simulink model "KUKAKR70"  (R2022b)
settings: Solver=ode4  StartTime=0.0  StopTime=SimulinkSimTime  FixedStep=Ts  RelTol=1e-3
values from neighbouring files (symbols this model uses):
  X = 1200    [KR70InverseDynamics.m]
  Y = 1200    [KR70InverseDynamics.m]
  Z = 1200    [KR70InverseDynamics.m]
libraries: nesl_utility x35, sm_lib x32, simulink_extras x7, sharedtransform x1
settings Model: Creator=Aboudi  LastModifiedBy=revdu
settings SolverCC: AlgebraicLoopSolver=TrustRegion
settings OptimizationCC: EnhancedBackFolding=on  PassReuseOutputArgsAs=Individual arguments  ZeroExternalMemoryAtStartup=off  ZeroInternalMemoryAtStartup=off  MaxStackSize=64  OptimizeBlockOrder=speed  DifferentSizesBufferReuse=on  OptimizationCustomize=off  EfficientTunableParamExpr=on
settings DebuggingCC: ParameterTunabilityLossMsg=error  UnconnectedInputMsg=warning  UnconnectedOutputMsg=warning  UnconnectedLineMsg=warning  SFMachineParentedDataDiag=warning
settings HardwareCC: ProdBitPerPointer=32  ProdBitPerSizeT=32  ProdBitPerPtrDiffT=32  ProdLargestAtomicFloat=None  ProdIntDivRoundTo=Undefined  ProdEndianess=Unspecified  ProdWordSize=32  ProdHWDeviceType=Generic->Unspecified (assume 32-bit Generic)
settings ModelReferenceCC: EnableRefExpFcnMdlSchedulingChecks=on
settings SFSimCC: MATLABDynamicMemAlloc=off
settings RTWCC: Description=Embedded Coder  SystemTargetFile=ert.tlc  HardwareBoard=Robot Operating System (ROS)  TLCOptions="-aInlineSetEventsForThisBaseRateFcn=TLC_FALSE -aSuppressMultiTaskScheduler=TLC_FALSE  -aRateBasedStepFcn=0"  TemplateMakefile=ert_default_tmf  Toolchain=Catkin  TargetLang=C++
settings CodeAppCC: ForceParamTrailComments=on  IgnoreCustomStorageClasses=off  OperatorAnnotations=on  SimulinkDataObjDesc=on  SFDataObjDesc=on  InsertBlockDesc=on
settings ExplorerConfigSet: InternalSimMechanicsExplorerSettings="<ExplorerConfiguration><canonicalview>aerospace</canonicalview><AnimationSetting><BasePlaybackSpeed>1.0</BasePlaybackSpeed><PlaybackSpeedFactor>1.0</PlaybackSpeedFactor></AnimationSetting><TilePanel><TileInfo><Tiles Columns=\"1\" Count=\"1\" Rows=\"1\"><Column Weight=\"1\"/><Row Weight=\"1\"/><Tile Height=\"1\" Width=\"1\" X=\"0\" Y=\"0\"/></Tiles></TileInfo><SceneInfo><SceneViewer><BGColor><R>0.60000002384185791</R><G>0.60000002384185791</G><B>0.60000002384185791</B></BGColor><Camera><DoPerspective>off</DoPerspective><Position><X>5.06313439550906796</X><Y>0.0784860108113666355</Y><Z>2.80097645569289577</Z></Position><Center><X>0.122639400059972203</X><Y>0.384687639263078585</Y><Z>0.502344850293265921</Z></Center><Up><X>-0.42040582822240502</X><Y>0.0254642749424247583</Y><Z>0.906978781614151353</Z></Up><ViewLimDist>1</ViewLimDist><YLim>1.2254397847778391</YLim><XLim>1.82716918582345955</XLim></Camera></SceneViewer></SceneInfo></TilePanel><MechEditorPanel><Cameras/><GfxPanelCameraMap/><VideoCreator><PlaybackSpeedRatio>1.0</PlaybackSpeedRatio><FrameRate>30</FrameRate><VideoFormat>Motion JPEG AVI</VideoFormat><FrameSize>auto</FrameSize></VideoCreator></MechEditorPanel></ExplorerConfiguration>"

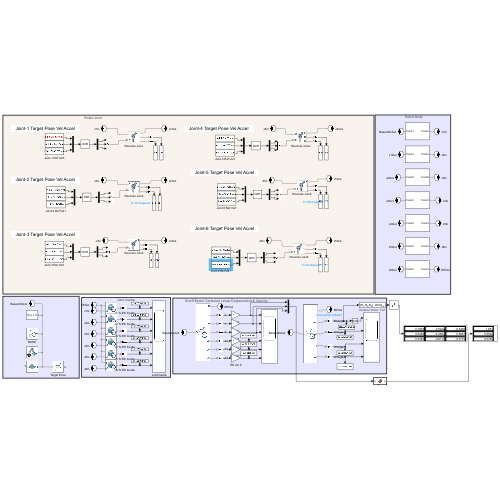
[thumbnail: Simulink's stored preview of the top-level diagram]
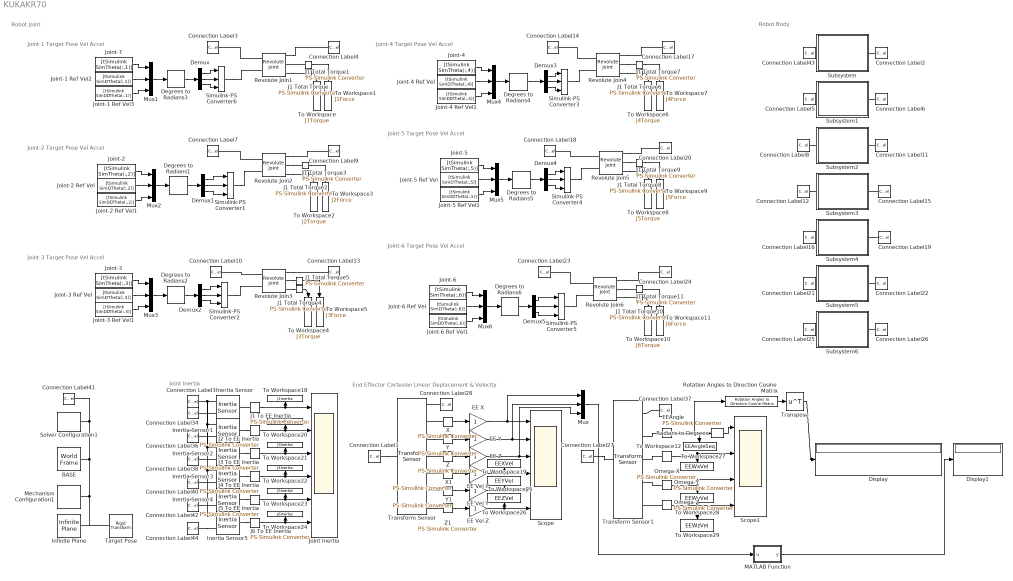
== system KUKAKR70 ==
  note: Robot Body
  note: Robot Joint
  note: Joint-1 Target Pose Vel Accel
  note: Joint-2 Target Pose Vel Accel
  note: Joint-3 Target Pose Vel Accel
  note: Joint-4 Target Pose Vel Accel
  note: Joint-5 Target Pose Vel Accel
  note: Joint-6 Target Pose Vel Accel
  note: Joint Inertia
  note: End Effector Cartesian Linear Deplacement & Velocity
  BASE : sm_lib/Frames and Transforms/World Frame
  Connection Label{1,27,41,43} (4 alike) : ConnectionLabel  Label=BasetoRobot
  Connection Label10 : ConnectionLabel  Label=J3In
  Connection Label11 : ConnectionLabel  Label=J3In
  Connection Label12 : ConnectionLabel  Label=J3Out
  Connection Label13 : ConnectionLabel  Label=J3Out
  Connection Label14 : ConnectionLabel  Label=J4In
  Connection Label15 : ConnectionLabel  Label=J4In
  Connection Label16 : ConnectionLabel  Label=J4Out
  Connection Label17 : ConnectionLabel  Label=J4Out
  Connection Label18 : ConnectionLabel  Label=J5In
  Connection Label19 : ConnectionLabel  Label=J5In
  Connection Label2 : ConnectionLabel  Label=J1In
  Connection Label20 : ConnectionLabel  Label=J5Out
  Connection Label21 : ConnectionLabel  Label=J5Out
  Connection Label22 : ConnectionLabel  Label=J6In
  Connection Label23 : ConnectionLabel  Label=J6In
  Connection Label24 : ConnectionLabel  Label=J6Out
  Connection Label25 : ConnectionLabel  Label=J6Out
  Connection Label{26,28,33,37} (4 alike) : ConnectionLabel  Label=EEOut
  Connection Label3 : ConnectionLabel  Label=J1In
  Connection Label34 : ConnectionLabel  Label=J1In
  Connection Label36 : ConnectionLabel  Label=J2In
  Connection Label38 : ConnectionLabel  Label=J3In
  Connection Label4 : ConnectionLabel  Label=J1Out
  Connection Label40 : ConnectionLabel  Label=J4In
  Connection Label42 : ConnectionLabel  Label=J5In
  Connection Label44 : ConnectionLabel  Label=J6In
  Connection Label5 : ConnectionLabel  Label=J1Out
  Connection Label6 : ConnectionLabel  Label=J2In
  Connection Label7 : ConnectionLabel  Label=J2In
  Connection Label8 : ConnectionLabel  Label=J2Out
  Connection Label9 : ConnectionLabel  Label=J2Out
  Degrees to Radians{1..6} (6 alike) : simulink_extras/Transformations/Degrees to Radians
  Demux{,1..5} (6 alike) : Demux  Outputs=3
  Display : Display
  Display1 : Display
  EE Vel X : Gain
  EE Vel Y : Gain
  EE Vel Z : Gain
  EE X : Gain
  EE Y : Gain
  EE Z : Gain
  EEAngle : nesl_utility/PS-Simulink Converter  PhysicalDomain=network_engine_domain  SubClassName=ps_output  LeftPortType=input  RightPortType=output  PseudoPeriodic=off  Frequencies=[]  VectorFormat=1-D array  Unit=rad  AffineConversion=off
  Inertia Sensor : sm_lib/Body Elements/Inertia Sensor  SensorExtent=BodyGroup  SpanWeldJoints=off  ExcludeGroundedBodies=off  MeasurementFrame=Custom  SenseMass=off  SenseCenterOfMass=off  SenseInertiaMatrix=on  SenseCenteredInertiaMatrix=off  SensePrincipalInertiaMatrix=off  SenseRotationMatrix=off  GraphicType=None  PrincipalInertiaFrameSize=20  GraphicVisPropType=SimpleVisualProperties  GraphicDiffuseColor=[1.0 1.0 0.0]  GraphicSpecularColor=[0.5 0.5 0.5 1.0]  GraphicAmbientColor=[0.15 0.15 0.15 1.0]  GraphicEmissiveColor=[0.0 0.0 0.0 1.0]  GraphicShininess=75  GraphicOpacity=0
  Inertia Sensor1 : sm_lib/Body Elements/Inertia Sensor  SensorExtent=BodyGroup  SpanWeldJoints=on  ExcludeGroundedBodies=off  MeasurementFrame=Custom  SenseMass=off  SenseCenterOfMass=off  SenseInertiaMatrix=on  SenseCenteredInertiaMatrix=off  SensePrincipalInertiaMatrix=off  SenseRotationMatrix=off  GraphicType=None  PrincipalInertiaFrameSize=20  GraphicVisPropType=SimpleVisualProperties  GraphicDiffuseColor=[1.0 1.0 0.0]  GraphicSpecularColor=[0.5 0.5 0.5 1.0]  GraphicAmbientColor=[0.15 0.15 0.15 1.0]  GraphicEmissiveColor=[0.0 0.0 0.0 1.0]  GraphicShininess=75  GraphicOpacity=1.0
  Inertia Sensor{2..5} (4 alike) : sm_lib/Body Elements/Inertia Sensor  SensorExtent=BodyGroup  SpanWeldJoints=off  ExcludeGroundedBodies=off  MeasurementFrame=Custom  SenseMass=off  SenseCenterOfMass=off  SenseInertiaMatrix=on  SenseCenteredInertiaMatrix=off  SensePrincipalInertiaMatrix=off  SenseRotationMatrix=off  GraphicType=None  PrincipalInertiaFrameSize=20  GraphicVisPropType=SimpleVisualProperties  GraphicDiffuseColor=[1.0 1.0 0.0]  GraphicSpecularColor=[0.5 0.5 0.5 1.0]  GraphicAmbientColor=[0.15 0.15 0.15 1.0]  GraphicEmissiveColor=[0.0 0.0 0.0 1.0]  GraphicShininess=75  GraphicOpacity=1.0
  Infinite Plane : sm_lib/Curves and Surfaces/Infinite Plane  GraphicType=Rectangle  GraphicPlaneWidth=5  GraphicPlaneWidthUnits=m  GraphicPlaneHeight=5  GraphicPlaneHeightUnits=m  GraphicVisPropType=SimpleVisualProperties  GraphicDiffuseColor=[1 0 0]  GraphicOpacity=.25  GraphicSpecularColor=[0.5 0.5 0.5 1.0]  GraphicAmbientColor=[0.15 0.15 0.15 1.0]  GraphicEmissiveColor=[0.0 0.0 0.0 1.0]  GraphicShininess=75
  J1 To EE Inertia : nesl_utility/PS-Simulink Converter  PhysicalDomain=network_engine_domain  SubClassName=ps_output  LeftPortType=input  RightPortType=output  PseudoPeriodic=off  Frequencies=[]  VectorFormat=1-D array  Unit=inherit  AffineConversion=off
  J1 Total Torque{,2,4,6,8,10} (6 alike) : nesl_utility/PS-Simulink Converter  PhysicalDomain=network_engine_domain  SubClassName=ps_output  LeftPortType=input  RightPortType=output  PseudoPeriodic=off  Frequencies=[]  VectorFormat=1-D array  Unit=N*m  AffineConversion=off
  J1 Total Torque{1,3,5,7,9,11} (6 alike) : nesl_utility/PS-Simulink Converter  PhysicalDomain=network_engine_domain  SubClassName=ps_output  LeftPortType=input  RightPortType=output  PseudoPeriodic=off  Frequencies=[]  VectorFormat=1-D array  Unit=N  AffineConversion=off
  J2 To EE Inertia : nesl_utility/PS-Simulink Converter  PhysicalDomain=network_engine_domain  SubClassName=ps_output  LeftPortType=input  RightPortType=output  PseudoPeriodic=off  Frequencies=[]  VectorFormat=1-D array  Unit=inherit  AffineConversion=off
  J3 To EE Inertia : nesl_utility/PS-Simulink Converter  PhysicalDomain=network_engine_domain  SubClassName=ps_output  LeftPortType=input  RightPortType=output  PseudoPeriodic=off  Frequencies=[]  VectorFormat=1-D array  Unit=inherit  AffineConversion=off
  J4 To EE Inertia : nesl_utility/PS-Simulink Converter  PhysicalDomain=network_engine_domain  SubClassName=ps_output  LeftPortType=input  RightPortType=output  PseudoPeriodic=off  Frequencies=[]  VectorFormat=1-D array  Unit=inherit  AffineConversion=off
  J5 To EE Inertia : nesl_utility/PS-Simulink Converter  PhysicalDomain=network_engine_domain  SubClassName=ps_output  LeftPortType=input  RightPortType=output  PseudoPeriodic=off  Frequencies=[]  VectorFormat=1-D array  Unit=inherit  AffineConversion=off
  J6 To EE Inertia : nesl_utility/PS-Simulink Converter  PhysicalDomain=network_engine_domain  SubClassName=ps_output  LeftPortType=input  RightPortType=output  PseudoPeriodic=off  Frequencies=[]  VectorFormat=1-D array  Unit=inherit  AffineConversion=off
  Joint Inertia : Scope  NumInputPorts=6
  Joint-1 Ref Vel2 : FromWorkspace  VariableName=[tSimulink SimDTheta(:,1)]  SampleTime=-1  OutputAfterFinalValue=Holding final value
  Joint-1 Ref Vel3 : FromWorkspace  VariableName=[tSimulink SimDDTheta(:,1)]  SampleTime=-1  OutputAfterFinalValue=Holding final value
  Joint-2 : FromWorkspace  VariableName=[tSimulink SimTheta(:,2)]  SampleTime=-1  OutputAfterFinalValue=Holding final value
  Joint-2 Ref Vel : FromWorkspace  VariableName=[tSimulink SimDTheta(:,2)]  SampleTime=-1  OutputAfterFinalValue=Holding final value
  Joint-2 Ref Vel1 : FromWorkspace  VariableName=[tSimulink SimDDTheta(:,2)]  SampleTime=-1  OutputAfterFinalValue=Holding final value
  Joint-3 : FromWorkspace  VariableName=[tSimulink SimTheta(:,3)]  SampleTime=-1  OutputAfterFinalValue=Holding final value
  Joint-3 Ref Vel : FromWorkspace  VariableName=[tSimulink SimDTheta(:,3)]  SampleTime=-1  OutputAfterFinalValue=Holding final value
  Joint-3 Ref Vel1 : FromWorkspace  VariableName=[tSimulink SimDDTheta(:,3)]  SampleTime=-1  OutputAfterFinalValue=Holding final value
  Joint-4 : FromWorkspace  VariableName=[tSimulink SimTheta(:,4)]  SampleTime=-1  OutputAfterFinalValue=Holding final value
  Joint-4 Ref Vel : FromWorkspace  VariableName=[tSimulink SimDTheta(:,4)]  SampleTime=-1  OutputAfterFinalValue=Holding final value
  Joint-4 Ref Vel1 : FromWorkspace  VariableName=[tSimulink SimDDTheta(:,4)]  SampleTime=-1  OutputAfterFinalValue=Holding final value
  Joint-5 : FromWorkspace  VariableName=[tSimulink SimTheta(:,5)]  SampleTime=-1  OutputAfterFinalValue=Holding final value
  Joint-5 Ref Vel : FromWorkspace  VariableName=[tSimulink SimDTheta(:,5)]  SampleTime=-1  OutputAfterFinalValue=Holding final value
  Joint-5 Ref Vel1 : FromWorkspace  VariableName=[tSimulink SimDDTheta(:,5)]  SampleTime=-1  OutputAfterFinalValue=Holding final value
  Joint-6 : FromWorkspace  VariableName=[tSimulink SimTheta(:,6)]  SampleTime=-1  OutputAfterFinalValue=Holding final value
  Joint-6 Ref Vel : FromWorkspace  VariableName=[tSimulink SimDTheta(:,6)]  SampleTime=-1  OutputAfterFinalValue=Holding final value
  Joint-6 Ref Vel1 : FromWorkspace  VariableName=[tSimulink SimDDTheta(:,6)]  SampleTime=-1  OutputAfterFinalValue=Holding final value
  Joint-7 : FromWorkspace  VariableName=[tSimulink SimTheta(:,1)]  SampleTime=-1  OutputAfterFinalValue=Holding final value
  MATLAB Function : MATLAB Function  TreatAsAtomicUnit=on
  Mechanism Configuration1 : sm_lib/Utilities/Mechanism Configuration  UniformGravity=Constant  GravityVector=[0 0 -9.80665]  GravityUnits=m/s^2  LinearizationDelta=0.001  JointModeTransitionNonlinearIterations=2
  Mux{,1..6} (7 alike) : Mux  Inputs=3
  Omega-X : nesl_utility/PS-Simulink Converter  PhysicalDomain=network_engine_domain  SubClassName=ps_output  LeftPortType=input  RightPortType=output  PseudoPeriodic=off  Frequencies=[]  VectorFormat=1-D array  Unit=rad/s  AffineConversion=off
  Omega-Y : nesl_utility/PS-Simulink Converter  PhysicalDomain=network_engine_domain  SubClassName=ps_output  LeftPortType=input  RightPortType=output  PseudoPeriodic=off  Frequencies=[]  VectorFormat=1-D array  Unit=rad/s  AffineConversion=off
  Omega-Z : nesl_utility/PS-Simulink Converter  PhysicalDomain=network_engine_domain  SubClassName=ps_output  LeftPortType=input  RightPortType=output  PseudoPeriodic=off  Frequencies=[]  VectorFormat=1-D array  Unit=rad/s  AffineConversion=off
  Radians to Degrees : simulink_extras/Transformations/Radians to Degrees
  Revolute Join{1..6} (6 alike) : sm_lib/Joints/Revolute Joint  JointMode=Normal  SenseConstraintForce=off  SenseConstraintForceX=off  SenseConstraintForceY=off  SenseConstraintForceZ=off  SenseConstraintTorque=off  SenseConstraintTorqueX=off  SenseConstraintTorqueY=off  SenseConstraintTorqueZ=off  SenseTotalForce=on  SenseTotalForceX=off  SenseTotalForceY=off  SenseTotalForceZ=off  SenseTotalTorque=on  SenseTotalTorqueX=off  SenseTotalTorqueY=off  SenseTotalTorqueZ=off  CompositeWrenchDir=FollowerOnBase  CompositeWrenchFrame=FollowerFrame  EquilibriumPosition=0  EquilibriumPositionUnits=deg  SpringStiffness=0  SpringStiffnessUnits=N*m/deg  DampingCoefficient=0  DampingCoefficientUnits=N*m/(deg/s)  TorqueActuationMode=ComputedTorque  MotionActuationMode=InputMotion  SensePosition=off  SenseVelocity=off  SenseAcceleration=off  SenseTorqueForce=off  SenseLowerLimitTorqueForce=off  SenseUpperLimitTorqueForce=off  LowerLimitSpecify=off  LowerLimitBound=-90  LowerLimitBoundUnits=deg  LowerLimitStiffness=1e4  LowerLimitStiffnessUnits=N*m/deg  LowerLimitDamping=10  LowerLimitDampingUnits=N*m/(deg/s)  LowerLimitTransitionRegionWidth=0.1  LowerLimitTransitionRegionWidthUnits=deg  UpperLimitSpecify=off  UpperLimitBound=90  UpperLimitBoundUnits=deg  UpperLimitStiffness=1e4  UpperLimitStiffnessUnits=N*m/deg  UpperLimitDamping=10  UpperLimitDampingUnits=N*m/(deg/s)  UpperLimitTransitionRegionWidth=0.1  UpperLimitTransitionRegionWidthUnits=deg  PositionTargetSpecify=off  PositionTargetPriority=High  PositionTargetValue=0  PositionTargetValueUnits=deg  VelocityTargetSpecify=off  VelocityTargetPriority=High  VelocityTargetValue=0  VelocityTargetValueUnits=deg/s
  Rotation Angles to Direction Cosine Matrix : sharedtransform/Rotation Angles to Direction Cosine Matrix  rotationOrder=XYZ  aMode=aMode
  Scope : Scope  NumInputPorts=6
  Scope1 : Scope  NumInputPorts=4
  Simulink-PS Converter{1..6} (6 alike) : nesl_utility/Simulink-PS Converter  PhysicalDomain=network_engine_domain  SubClassName=ps_input  LeftPortType=input  RightPortType=output  PseudoPeriodic=off  Frequencies=[]  NoiseDistribution=none  NoiseParameters=[]  Unit=1  AffineConversion=off  FilteringAndDerivatives=provide  SimscapeFilterOrder=2  InputFilterTimeConstant=Ts  UdotUserProvided=2
  Solver Configuration1 : nesl_utility/Solver Configuration  PhysicalDomain=network_engine_domain  SubClassName=solver  LeftPortType=input  RightPortType=generic  Tones=[]  Harmonics=[]  SimulateNoise=off  Profile=off  UseLocalSampling=off  EnableSwitchedLinearOptims=on  FrequencyDomain=off  UseCCode=off  RelTol=0.001  AbsTol=1e-06  MinStep=1e-09  ToWorkspace=off  RevertToSquareIcSolve=off  NumHomotopyIterations=100  PhasorMode=off  PhasorModeNumHarmonics=1  ConsistencySolver=NEWTON_FTOL  IndexReductionMethod=DerivativeReplacement  DoDC=off  ResidualTolerance=1e-09  ConsistencyTolSource=GLOBAL  ConsistencyAbsTol=0.001  ConsistencyRelTol=0.001  ConsistencyTolFactor=0.001  UseLocalSolver=off  LocalSolverChoice=NE_BACKWARD_EULER_ADVANCER  ResolveIndetEquations=on  FunctionEvalNumThread=1  LocalSolverSampleTime=0.001  DoFixedCost=off  MaxNonlinIter=3  MaxModeIter=2  ComputeImpulses=off  ImpulseIterations=2  LinearAlgebra=Full  LinearAlgebraNumThread=0  EquationFormulation=NE_FREQUENCY_TIME_EF  DelaysMemoryBudget=1024  AutomaticFiltering=on  FilteringTimeConstant=0.001  PartitionStorageMethod=AS_NEEDED  PartitionMemoryBudget=1024  PartitionMethod=FAST
  Subsystem : Subsystem
  Subsystem1 : Subsystem
  Subsystem2 : Subsystem
  Subsystem3 : Subsystem
  Subsystem4 : Subsystem
  Subsystem5 : Subsystem
  Subsystem6 : Subsystem
  Target Pose : sm_lib/Frames and Transforms/Rigid Transform  TranslationMethod=Cartesian  TranslationStandardOffset=0  TranslationLengthUnit=mm  TranslationStandardAxis=+Z  TranslationCartesianOffset=AllTargetPose(1:3,4,end)  TranslationROffset=0  TranslationROffsetUnits=m  TranslationZOffset=0  TranslationZOffsetUnits=m  TranslationThetaOffset=0  TranslationThetaOffsetUnits=deg  RotationMethod=RotationMatrix  RotationAngleUnits=deg  RotationStandardAxis=+Z  RotationAngle=0.0  RotationArbitraryAxis=[0 0 1]  FollAlignAxisA=+X  BaseAlignAxisA=+Y  FollAlignAxisB=+Y  BaseAlignAxisB=+Z  RotationSequenceAxes=FollowerAxes  RotationSequence=XYX  RotationSequenceAngles=[0 0 0]  RotationSequenceAnglesUnits=deg  RotationMatrix=AllTargetPose(1:3,1:3,end)  Quaternion=[1 0 0 0]
  To Workspace : ToWorkspace  VariableName=J1Torque  SaveFormat=Timeseries  SampleTime=-1
  To Workspace1 : ToWorkspace  VariableName=J1Force  SaveFormat=Timeseries  SampleTime=-1
  To Workspace10 : ToWorkspace  VariableName=J6Torque  SaveFormat=Timeseries  SampleTime=-1
  To Workspace11 : ToWorkspace  VariableName=J6Force  SaveFormat=Timeseries  SampleTime=-1
  To Workspace12 : ToWorkspace  VariableName=EEAngleSeq  SaveFormat=Timeseries  SampleTime=-1
  To Workspace18 : ToWorkspace  VariableName=J1Inertia  SaveFormat=Timeseries  SampleTime=-1
  To Workspace19 : ToWorkspace  VariableName=EEXVel  SaveFormat=Timeseries  SampleTime=-1
  To Workspace2 : ToWorkspace  VariableName=J2Torque  SaveFormat=Timeseries  SampleTime=-1
  To Workspace20 : ToWorkspace  VariableName=J2Inertia  SaveFormat=Timeseries  SampleTime=-1
  To Workspace21 : ToWorkspace  VariableName=J3Inertia  SaveFormat=Timeseries  SampleTime=-1
  To Workspace22 : ToWorkspace  VariableName=J4Inertia  SaveFormat=Timeseries  SampleTime=-1
  To Workspace23 : ToWorkspace  VariableName=J5Inertia  SaveFormat=Timeseries  SampleTime=-1
  To Workspace24 : ToWorkspace  VariableName=J6Inertia  SaveFormat=Timeseries  SampleTime=-1
  To Workspace25 : ToWorkspace  VariableName=EEYVel  SaveFormat=Timeseries  SampleTime=-1
  To Workspace26 : ToWorkspace  VariableName=EEZVel  SaveFormat=Timeseries  SampleTime=-1
  To Workspace27 : ToWorkspace  VariableName=EEWxVel  SaveFormat=Timeseries  SampleTime=-1
  To Workspace28 : ToWorkspace  VariableName=EEWyVel  SaveFormat=Timeseries  SampleTime=-1
  To Workspace29 : ToWorkspace  VariableName=EEWzVel  SaveFormat=Timeseries  SampleTime=-1
  To Workspace3 : ToWorkspace  VariableName=J2Force  SaveFormat=Timeseries  SampleTime=-1
  To Workspace4 : ToWorkspace  VariableName=J3Torque  SaveFormat=Timeseries  SampleTime=-1
  To Workspace5 : ToWorkspace  VariableName=J3Force  SaveFormat=Timeseries  SampleTime=-1
  To Workspace6 : ToWorkspace  VariableName=J4Torque  SaveFormat=Timeseries  SampleTime=-1
  To Workspace7 : ToWorkspace  VariableName=J4Force  SaveFormat=Timeseries  SampleTime=-1
  To Workspace8 : ToWorkspace  VariableName=J5Torque  SaveFormat=Timeseries  SampleTime=-1
  To Workspace9 : ToWorkspace  VariableName=J5Force  SaveFormat=Timeseries  SampleTime=-1
  Transform Sensor : sm_lib/Frames and Transforms/Transform Sensor  MeasurementFrame=World  SenseAngle=off  SenseAxis=off  SenseQ=off  SenseR=off  SenseRotationSequence=off  RotationSequence=XYX  SenseOmegaX=off  SenseOmegaY=off  SenseOmegaZ=off  SenseQDot=off  SenseRDot=off  SenseAlphaX=off  SenseAlphaY=off  SenseAlphaZ=off  SenseQDDot=off  SenseRDDot=off  SenseX=on  SenseY=on  SenseZ=on  SenseRad=off  SenseAzim=off  SenseDist=off  SenseInc=off  SenseXDot=on  SenseYDot=on  SenseZDot=on  SenseRadDot=off  SenseAzimDot=off  SenseDistDot=off  SenseIncDot=off  SenseXDDot=off  SenseYDDot=off  SenseZDDot=off  SenseRadDDot=off  SenseAzimDDot=off  SenseDistDDot=off  SenseIncDDot=off
  Transform Sensor1 : sm_lib/Frames and Transforms/Transform Sensor  MeasurementFrame=World  SenseAngle=off  SenseAxis=off  SenseQ=off  SenseR=off  SenseRotationSequence=on  RotationSequence=XYZ  SenseOmegaX=on  SenseOmegaY=on  SenseOmegaZ=on  SenseQDot=off  SenseRDot=off  SenseAlphaX=off  SenseAlphaY=off  SenseAlphaZ=off  SenseQDDot=off  SenseRDDot=off  SenseX=off  SenseY=off  SenseZ=off  SenseRad=off  SenseAzim=off  SenseDist=off  SenseInc=off  SenseXDot=off  SenseYDot=off  SenseZDot=off  SenseRadDot=off  SenseAzimDot=off  SenseDistDot=off  SenseIncDot=off  SenseXDDot=off  SenseYDDot=off  SenseZDDot=off  SenseRadDDot=off  SenseAzimDDot=off  SenseDistDDot=off  SenseIncDDot=off
  Transpose : Math  Operator=transpose
  X : nesl_utility/PS-Simulink Converter  PhysicalDomain=network_engine_domain  SubClassName=ps_output  LeftPortType=input  RightPortType=output  PseudoPeriodic=off  Frequencies=[]  VectorFormat=1-D array  Unit=m  AffineConversion=off
  X1 : nesl_utility/PS-Simulink Converter  PhysicalDomain=network_engine_domain  SubClassName=ps_output  LeftPortType=input  RightPortType=output  PseudoPeriodic=off  Frequencies=[]  VectorFormat=1-D array  Unit=m/s  AffineConversion=off
  Y : nesl_utility/PS-Simulink Converter  PhysicalDomain=network_engine_domain  SubClassName=ps_output  LeftPortType=input  RightPortType=output  PseudoPeriodic=off  Frequencies=[]  VectorFormat=1-D array  Unit=m  AffineConversion=off
  Y1 : nesl_utility/PS-Simulink Converter  PhysicalDomain=network_engine_domain  SubClassName=ps_output  LeftPortType=input  RightPortType=output  PseudoPeriodic=off  Frequencies=[]  VectorFormat=1-D array  Unit=m/s  AffineConversion=off
  Z : nesl_utility/PS-Simulink Converter  PhysicalDomain=network_engine_domain  SubClassName=ps_output  LeftPortType=input  RightPortType=output  PseudoPeriodic=off  Frequencies=[]  VectorFormat=1-D array  Unit=m  AffineConversion=off
  Z1 : nesl_utility/PS-Simulink Converter  PhysicalDomain=network_engine_domain  SubClassName=ps_output  LeftPortType=input  RightPortType=output  PseudoPeriodic=off  Frequencies=[]  VectorFormat=1-D array  Unit=m/s  AffineConversion=off
  wires:
  Joint-1 Ref Vel2/1 -> Mux1/2
  Joint-7/1 -> Mux1/1
  Joint-1 Ref Vel3/1 -> Mux1/3
  Mux1/1 -> Degrees to Radians3/1
  Degrees to Radians3/1 -> Demux/1
  Demux/1 -> Simulink-PS Converter6/1
  Demux/2 -> Simulink-PS Converter6/2
  Demux/3 -> Simulink-PS Converter6/3
  Demux1/3 -> Simulink-PS Converter1/3
  Demux1/2 -> Simulink-PS Converter1/2
  Demux1/1 -> Simulink-PS Converter1/1
  Degrees to Radians1/1 -> Demux1/1
  Mux2/1 -> Degrees to Radians1/1
  Joint-2 Ref Vel1/1 -> Mux2/3
  Joint-2/1 -> Mux2/1
  Joint-2 Ref Vel/1 -> Mux2/2
  Joint-3 Ref Vel/1 -> Mux3/2
  Joint-3/1 -> Mux3/1
  Joint-3 Ref Vel1/1 -> Mux3/3
  Mux3/1 -> Degrees to Radians2/1
  Degrees to Radians2/1 -> Demux2/1
  Demux2/1 -> Simulink-PS Converter2/1
  Demux2/2 -> Simulink-PS Converter2/2
  Demux2/3 -> Simulink-PS Converter2/3
  Joint-4/1 -> Mux4/1
  Demux3/3 -> Simulink-PS Converter3/3
  Demux3/1 -> Simulink-PS Converter3/1
  Degrees to Radians4/1 -> Demux3/1
  Joint-4 Ref Vel1/1 -> Mux4/3
  Demux3/2 -> Simulink-PS Converter3/2
  Mux4/1 -> Degrees to Radians4/1
  Joint-4 Ref Vel/1 -> Mux4/2
  Demux4/3 -> Simulink-PS Converter4/3
  Demux4/2 -> Simulink-PS Converter4/2
  Demux4/1 -> Simulink-PS Converter4/1
  Degrees to Radians5/1 -> Demux4/1
  Mux5/1 -> Degrees to Radians5/1
  Joint-5 Ref Vel1/1 -> Mux5/3
  Joint-5/1 -> Mux5/1
  Joint-5 Ref Vel/1 -> Mux5/2
  Joint-6 Ref Vel/1 -> Mux6/2
  Joint-6/1 -> Mux6/1
  Joint-6 Ref Vel1/1 -> Mux6/3
  Mux6/1 -> Degrees to Radians6/1
  Degrees to Radians6/1 -> Demux5/1
  Demux5/1 -> Simulink-PS Converter5/1
  Demux5/2 -> Simulink-PS Converter5/2
  Demux5/3 -> Simulink-PS Converter5/3
  J1 Total Torque/1 -> To Workspace/1
  J1 Total Torque1/1 -> To Workspace1/1
  J1 Total Torque3/1 -> To Workspace3/1
  J1 Total Torque2/1 -> To Workspace2/1
  J1 Total Torque4/1 -> To Workspace4/1
  J1 Total Torque5/1 -> To Workspace5/1
  J1 Total Torque7/1 -> To Workspace7/1
  J1 Total Torque6/1 -> To Workspace6/1
  J1 Total Torque8/1 -> To Workspace8/1
  J1 Total Torque9/1 -> To Workspace9/1
  J1 Total Torque11/1 -> To Workspace11/1
  J1 Total Torque10/1 -> To Workspace10/1
  J2 To EE Inertia/1 -> To Workspace20/1, Joint Inertia/2
  J1 To EE Inertia/1 -> To Workspace18/1, Joint Inertia/1
  J3 To EE Inertia/1 -> To Workspace21/1, Joint Inertia/3
  J6 To EE Inertia/1 -> To Workspace24/1, Joint Inertia/6
  J5 To EE Inertia/1 -> To Workspace23/1, Joint Inertia/5
  J4 To EE Inertia/1 -> To Workspace22/1, Joint Inertia/4
  EE Vel X/1 -> Scope/4, To Workspace19/1
  EE X/1 -> Mux/1, Scope/1
  EE Vel Z/1 -> To Workspace26/1, Scope/6
  Z1/1 -> EE Vel Z/1
  Z/1 -> EE Z/1
  EE Z/1 -> Mux/3, Scope/3
  Y1/1 -> EE Vel Y/1
  EE Y/1 -> Mux/2, Scope/2
  Y/1 -> EE Y/1
  X/1 -> EE X/1
  EE Vel Y/1 -> To Workspace25/1, Scope/5
  Omega-Z/1 -> To Workspace29/1, Scope1/4
  X1/1 -> EE Vel X/1
  Omega-Y/1 -> Scope1/3, To Workspace28/1
  Omega-X/1 -> Scope1/2, To Workspace27/1
  EEAngle/1 -> Rotation Angles to Direction Cosine Matrix/1, To Workspace12/1, Radians to Degrees/1
  Radians to Degrees/1 -> Scope1/1
  Rotation Angles to Direction Cosine Matrix/1 -> Transpose/1
  Mux/1 -> MATLAB Function/1(u)
  MATLAB Function/1(y) -> Display1/1
  Transpose/1 -> Display/1
  connections:
  Mechanism Configuration1/RConn1 -- Solver Configuration1/RConn1 -- Connection Label41/LConn1 -- BASE/RConn1 -- Target Pose/LConn1 -- Infinite Plane/LConn1
  Revolute Join5/RConn1 -- Connection Label20/LConn1
  Connection Label19/LConn1 -- Subsystem4/RConn1
  Subsystem3/LConn1 -- Connection Label12/LConn1
  Connection Label25/LConn1 -- Subsystem6/LConn1
  Revolute Join2/LConn1 -- Connection Label7/LConn1
  Revolute Join3/RConn1 -- Connection Label13/LConn1
  Connection Label15/LConn1 -- Subsystem3/RConn1
  Revolute Join1/LConn1 -- Connection Label3/LConn1
  Connection Label21/LConn1 -- Subsystem5/LConn1
  Connection Label16/LConn1 -- Subsystem4/LConn1
  Revolute Join2/RConn1 -- Connection Label9/LConn1
  Revolute Join5/LConn1 -- Connection Label18/LConn1
  Connection Label5/LConn1 -- Subsystem1/LConn1
  Revolute Join6/RConn1 -- Connection Label24/LConn1
  Connection Label11/LConn1 -- Subsystem2/RConn1
  Revolute Join6/LConn1 -- Connection Label23/LConn1
  Revolute Join3/LConn1 -- Connection Label10/LConn1
  Connection Label22/LConn1 -- Subsystem5/RConn1
  Revolute Join4/LConn1 -- Connection Label14/LConn1
  Connection Label2/LConn1 -- Subsystem/RConn1
  Connection Label43/LConn1 -- Subsystem/LConn1
  Revolute Join1/RConn1 -- Connection Label4/LConn1
  Connection Label6/LConn1 -- Subsystem1/RConn1
  Subsystem2/LConn1 -- Connection Label8/LConn1
  Connection Label26/LConn1 -- Subsystem6/RConn1
  Revolute Join4/RConn1 -- Connection Label17/LConn1
  Simulink-PS Converter6/RConn1 -- Revolute Join1/LConn2
  Simulink-PS Converter1/RConn1 -- Revolute Join2/LConn2
  Simulink-PS Converter2/RConn1 -- Revolute Join3/LConn2
  Simulink-PS Converter3/RConn1 -- Revolute Join4/LConn2
  Simulink-PS Converter4/RConn1 -- Revolute Join5/LConn2
  Simulink-PS Converter5/RConn1 -- Revolute Join6/LConn2
  Revolute Join1/RConn3 -- J1 Total Torque/LConn1
  J1 Total Torque1/LConn1 -- Revolute Join1/RConn2
  Revolute Join2/RConn2 -- J1 Total Torque3/LConn1
  Revolute Join2/RConn3 -- J1 Total Torque2/LConn1
  Revolute Join3/RConn3 -- J1 Total Torque4/LConn1
  Revolute Join3/RConn2 -- J1 Total Torque5/LConn1
  Revolute Join4/RConn2 -- J1 Total Torque7/LConn1
  Revolute Join4/RConn3 -- J1 Total Torque6/LConn1
  Revolute Join5/RConn3 -- J1 Total Torque8/LConn1
  Revolute Join5/RConn2 -- J1 Total Torque9/LConn1
  Revolute Join6/RConn3 -- J1 Total Torque10/LConn1
  Revolute Join6/RConn2 -- J1 Total Torque11/LConn1
  Connection Label33/LConn1 -- Inertia Sensor1/LConn1 -- Inertia Sensor2/LConn1 -- Inertia Sensor4/LConn1 -- Inertia Sensor5/LConn1 -- Inertia Sensor3/LConn1 -- Inertia Sensor/LConn1
  Connection Label34/LConn1 -- Inertia Sensor/LConn2
  Connection Label38/LConn1 -- Inertia Sensor2/LConn2
  Inertia Sensor3/RConn1 -- J4 To EE Inertia/LConn1
  Inertia Sensor1/RConn1 -- J2 To EE Inertia/LConn1
  J1 To EE Inertia/LConn1 -- Inertia Sensor/RConn1
  Connection Label40/LConn1 -- Inertia Sensor3/LConn2
  Inertia Sensor5/RConn1 -- J6 To EE Inertia/LConn1
  Connection Label42/LConn1 -- Inertia Sensor4/LConn2
  Connection Label36/LConn1 -- Inertia Sensor1/LConn2
  Inertia Sensor4/RConn1 -- J5 To EE Inertia/LConn1
  Connection Label44/LConn1 -- Inertia Sensor5/LConn2
  Inertia Sensor2/RConn1 -- J3 To EE Inertia/LConn1
  X/LConn1 -- Transform Sensor/RConn2
  Connection Label1/LConn1 -- Transform Sensor/LConn1
  X1/LConn1 -- Transform Sensor/RConn5
  Transform Sensor/RConn3 -- Y/LConn1
  Z1/LConn1 -- Transform Sensor/RConn7
  Connection Label27/LConn1 -- Transform Sensor1/LConn1
  Z/LConn1 -- Transform Sensor/RConn4
  Y1/LConn1 -- Transform Sensor/RConn6
  Connection Label37/LConn1 -- Transform Sensor1/RConn1
  Connection Label28/LConn1 -- Transform Sensor/RConn1
  Omega-Z/LConn1 -- Transform Sensor1/RConn5
  Omega-Y/LConn1 -- Transform Sensor1/RConn4
  Omega-X/LConn1 -- Transform Sensor1/RConn3
  EEAngle/LConn1 -- Transform Sensor1/RConn2

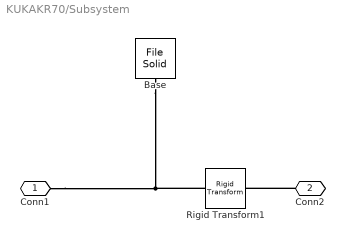
== system KUKAKR70/Subsystem ==
  Base : sm_lib/Body Elements/File Solid  ExtGeomFileName=C:\Users\revdu\OneDrive\Belgeler\GitHub\KukaKR70KinematicDynamicAnalysis\ComputedTorqueControl\stl\base.STL  UnitType=Custom  ExtGeomFileUnits=mm  StepReaderType=HEX  ExportConvexHullGeometry=off  InertiaType=Custom  Mass=92.377  MassUnits=kg  CenterOfMass=[-81.70 0.37 86.92]  CenterOfMassUnits=mm  MomentsOfInertia=[1.903 4.034 3.964]  MomentsOfInertiaUnits=kg*m^2  ProductsOfInertia=[-0.010 -0.853 0.003]  ProductsOfInertiaUnits=kg*m^2  BasedOnType=Mass  Density=3060.27  DensityUnits=kg/m^3  DoExposeReferenceFrame=on  SerializedFrames=<Frames/>  GraphicType=FromGeometry  MarkerShape=Frame  MarkerSize=10  GraphicVisPropType=SimpleVisualProperties  GraphicDiffuseColor=[0.4 0.4 0.4]  GraphicSpecularColor=[0.5 0.5 0.5 1.0]  GraphicAmbientColor=[0.15 0.15 0.15 1.0]  GraphicEmissiveColor=[0.0 0.0 0.0 1.0]  GraphicShininess=75  GraphicOpacity=1.0
  Rigid Transform1 : sm_lib/Frames and Transforms/Rigid Transform  TranslationMethod=Cartesian  TranslationStandardOffset=0  TranslationLengthUnit=mm  TranslationStandardAxis=+Z  TranslationCartesianOffset=[0 0 180]  TranslationROffset=0  TranslationROffsetUnits=m  TranslationZOffset=0  TranslationZOffsetUnits=m  TranslationThetaOffset=0  TranslationThetaOffsetUnits=deg  RotationMethod=ArbitraryAxis  RotationAngleUnits=deg  RotationStandardAxis=+Z  RotationAngle=0  RotationArbitraryAxis=[1 0 0]  FollAlignAxisA=+X  BaseAlignAxisA=+Y  FollAlignAxisB=+Y  BaseAlignAxisB=+Z  RotationSequenceAxes=FollowerAxes  RotationSequence=XYX  RotationSequenceAngles=[0 0 0]  RotationSequenceAnglesUnits=deg  RotationMatrix=[1 0 0; 0 1 0; 0 0 1]  Quaternion=[1 0 0 0]
  Conn1 : PMIOPort  Side=Left
  Conn2 : PMIOPort  Port=2  Side=Right
  connections:
  Base/RConn1 -- Rigid Transform1/LConn1 -- Conn1/RConn1
  Conn2/RConn1 -- Rigid Transform1/RConn1

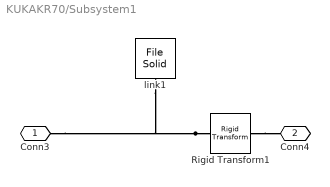
== system KUKAKR70/Subsystem1 ==
  Rigid Transform1 : sm_lib/Frames and Transforms/Rigid Transform  TranslationMethod=Cartesian  TranslationStandardOffset=0  TranslationLengthUnit=mm  TranslationStandardAxis=+Z  TranslationCartesianOffset=[175 -116.5 395]  TranslationROffset=0  TranslationROffsetUnits=m  TranslationZOffset=0  TranslationZOffsetUnits=m  TranslationThetaOffset=0  TranslationThetaOffsetUnits=deg  RotationMethod=RotationSequence  RotationAngleUnits=deg  RotationStandardAxis=+X  RotationAngle=90  RotationArbitraryAxis=[1 0 0]  FollAlignAxisA=+X  BaseAlignAxisA=+Y  FollAlignAxisB=+Y  BaseAlignAxisB=+Z  RotationSequenceAxes=FollowerAxes  RotationSequence=XYZ  RotationSequenceAngles=[90 0 0]  RotationSequenceAnglesUnits=deg  RotationMatrix=[1 0 0; 0 1 0; 0 0 1]  Quaternion=[1 0 0 0]
  link1 : sm_lib/Body Elements/File Solid  ExtGeomFileName=C:\Users\revdu\OneDrive\Belgeler\GitHub\KukaKR70KinematicDynamicAnalysis\ComputedTorqueControl\stl\link1.stl  UnitType=Custom  ExtGeomFileUnits=mm  StepReaderType=HEX  ExportConvexHullGeometry=off  InertiaType=Custom  Mass=171.666  MassUnits=kg  CenterOfMass=[60.05 11.67 237.06]  CenterOfMassUnits=mm  MomentsOfInertia=[14.911 16.857 4.672]  MomentsOfInertiaUnits=kg*m^2  ProductsOfInertia=[0.056 4.051 0.571]  ProductsOfInertiaUnits=kg*m^2  BasedOnType=DensityFromFile  Density=1000  DensityUnits=kg/m^3  DoExposeReferenceFrame=on  SerializedFrames=<Frames/>  GraphicType=FromGeometry  MarkerShape=Sphere  MarkerSize=10  GraphicVisPropType=SimpleVisualProperties  GraphicDiffuseColor=[1.0 0.6 0.2]  GraphicSpecularColor=[0.5 0.5 0.5 1.0]  GraphicAmbientColor=[0.15 0.15 0.15 1.0]  GraphicEmissiveColor=[0.0 0.0 0.0 1.0]  GraphicShininess=75  GraphicOpacity=1.0
  Conn3 : PMIOPort  Side=Left
  Conn4 : PMIOPort  Port=2  Side=Right
  connections:
  Rigid Transform1/LConn1 -- Conn3/RConn1 -- link1/RConn1
  Rigid Transform1/RConn1 -- Conn4/RConn1

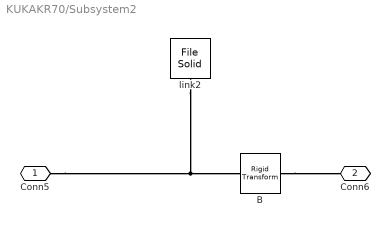
== system KUKAKR70/Subsystem2 ==
  B : sm_lib/Frames and Transforms/Rigid Transform  TranslationMethod=Cartesian  TranslationStandardOffset=0  TranslationLengthUnit=mm  TranslationStandardAxis=+Z  TranslationCartesianOffset=[890 0 63]  TranslationROffset=0  TranslationROffsetUnits=m  TranslationZOffset=0  TranslationZOffsetUnits=m  TranslationThetaOffset=0  TranslationThetaOffsetUnits=deg  RotationMethod=RotationSequence  RotationAngleUnits=deg  RotationStandardAxis=-Z  RotationAngle=90  RotationArbitraryAxis=[1 0 1]  FollAlignAxisA=+X  BaseAlignAxisA=+Y  FollAlignAxisB=+Y  BaseAlignAxisB=+Z  RotationSequenceAxes=FollowerAxes  RotationSequence=XYZ  RotationSequenceAngles=[0 0 0]  RotationSequenceAnglesUnits=deg  RotationMatrix=[1 0 0; 0 1 0; 0 0 1]  Quaternion=[1 0 0 0]
  link2 : sm_lib/Body Elements/File Solid  ExtGeomFileName=C:\Users\revdu\OneDrive\Belgeler\GitHub\KukaKR70KinematicDynamicAnalysis\ComputedTorqueControl\stl\link2.stl  UnitType=Custom  ExtGeomFileUnits=mm  StepReaderType=HEX  ExportConvexHullGeometry=off  InertiaType=Custom  Mass=61.522  MassUnits=kg  CenterOfMass=[401.52 -2.70 114.34]  CenterOfMassUnits=mm  MomentsOfInertia=[1.2 14.821 14.09]  MomentsOfInertiaUnits=kg*m^2  ProductsOfInertia=[0.009 3.165 -0.015]  ProductsOfInertiaUnits=kg*m^2  BasedOnType=DensityFromFile  Density=1000  DensityUnits=kg/m^3  DoExposeReferenceFrame=on  SerializedFrames=<Frames/>  GraphicType=FromGeometry  MarkerShape=Sphere  MarkerSize=10  GraphicVisPropType=SimpleVisualProperties  GraphicDiffuseColor=[1.0 0.6 0.2]  GraphicSpecularColor=[0.5 0.5 0.5 1.0]  GraphicAmbientColor=[0.15 0.15 0.15 1.0]  GraphicEmissiveColor=[0.0 0.0 0.0 1.0]  GraphicShininess=75  GraphicOpacity=1.0
  Conn5 : PMIOPort  Side=Left
  Conn6 : PMIOPort  Port=2  Side=Right
  connections:
  B/RConn1 -- Conn6/RConn1
  Conn5/RConn1 -- B/LConn1 -- link2/RConn1

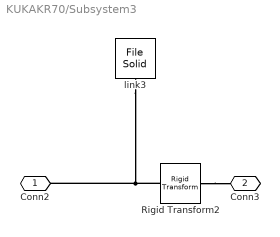
== system KUKAKR70/Subsystem3 ==
  Rigid Transform2 : sm_lib/Frames and Transforms/Rigid Transform  TranslationMethod=Cartesian  TranslationStandardOffset=0  TranslationLengthUnit=mm  TranslationStandardAxis=+Z  TranslationCartesianOffset="[50 -346.75  -179.5]"  TranslationROffset=0  TranslationROffsetUnits=m  TranslationZOffset=0  TranslationZOffsetUnits=m  TranslationThetaOffset=0  TranslationThetaOffsetUnits=deg  RotationMethod=RotationSequence  RotationAngleUnits=deg  RotationStandardAxis=+Z  RotationAngle=0.0  RotationArbitraryAxis=[0 0 1]  FollAlignAxisA=+X  BaseAlignAxisA=+Y  FollAlignAxisB=+Y  BaseAlignAxisB=+Z  RotationSequenceAxes=FollowerAxes  RotationSequence=XYZ  RotationSequenceAngles=[90 0 0]  RotationSequenceAnglesUnits=deg  RotationMatrix=[1 0 0; 0 1 0; 0 0 1]  Quaternion=[1 0 0 0]
  link3 : sm_lib/Body Elements/File Solid  ExtGeomFileName=C:\Users\revdu\OneDrive\Belgeler\GitHub\KukaKR70KinematicDynamicAnalysis\ComputedTorqueControl\stl\link3.stl  UnitType=Custom  ExtGeomFileUnits=mm  StepReaderType=HEX  ExportConvexHullGeometry=off  InertiaType=Custom  Mass=112.262  MassUnits=kg  CenterOfMass=[16.22 -30.50 -201.80]  CenterOfMassUnits=mm  MomentsOfInertia=[7.783 6.632 2.542]  MomentsOfInertiaUnits=kg*m^2  ProductsOfInertia=[-0.307 -0.0356 0.493]  ProductsOfInertiaUnits=kg*m^2  BasedOnType=DensityFromFile  Density=1000  DensityUnits=kg/m^3  DoExposeReferenceFrame=on  SerializedFrames=<Frames/>  GraphicType=FromGeometry  MarkerShape=Cube  MarkerSize=10  GraphicVisPropType=SimpleVisualProperties  GraphicDiffuseColor=[0.4 0.4 0.4]  GraphicSpecularColor=[0.5 0.5 0.5 1.0]  GraphicAmbientColor=[0.15 0.15 0.15 1.0]  GraphicEmissiveColor=[0.0 0.0 0.0 1.0]  GraphicShininess=75  GraphicOpacity=1.0
  Conn2 : PMIOPort  Side=Left
  Conn3 : PMIOPort  Port=2  Side=Right
  connections:
  Rigid Transform2/RConn1 -- Conn3/RConn1
  Rigid Transform2/LConn1 -- Conn2/RConn1 -- link3/RConn1

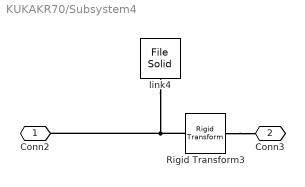
== system KUKAKR70/Subsystem4 ==
  Rigid Transform3 : sm_lib/Frames and Transforms/Rigid Transform  TranslationMethod=Cartesian  TranslationStandardOffset=0  TranslationLengthUnit=mm  TranslationStandardAxis=+Z  TranslationCartesianOffset=[0 0 688.25]  TranslationROffset=0  TranslationROffsetUnits=m  TranslationZOffset=0  TranslationZOffsetUnits=m  TranslationThetaOffset=0  TranslationThetaOffsetUnits=deg  RotationMethod=RotationSequence  RotationAngleUnits=deg  RotationStandardAxis=+Z  RotationAngle=0.0  RotationArbitraryAxis=[0 0 1]  FollAlignAxisA=+X  BaseAlignAxisA=+Y  FollAlignAxisB=+Y  BaseAlignAxisB=+Z  RotationSequenceAxes=FollowerAxes  RotationSequence=XYZ  RotationSequenceAngles=[-90 0 0]  RotationSequenceAnglesUnits=deg  RotationMatrix=[1 0 0; 0 1 0; 0 0 1]  Quaternion=[1 0 0 0]
  link4 : sm_lib/Body Elements/File Solid  ExtGeomFileName=C:\Users\revdu\OneDrive\Belgeler\GitHub\KukaKR70KinematicDynamicAnalysis\ComputedTorqueControl\stl\link4.stl  UnitType=Custom  ExtGeomFileUnits=mm  StepReaderType=HEX  ExportConvexHullGeometry=off  InertiaType=Custom  Mass=46.376  MassUnits=kg  CenterOfMass=[-0.06 -28.06 380.21]  CenterOfMassUnits=mm  MomentsOfInertia=[9.031 8.938 0.251]  MomentsOfInertiaUnits=kg*m^2  ProductsOfInertia=[0.0 -0.002 -0.798]  ProductsOfInertiaUnits=kg*m^2  BasedOnType=DensityFromFile  Density=1000  DensityUnits=kg/m^3  DoExposeReferenceFrame=on  SerializedFrames=<Frames/>  GraphicType=FromGeometry  MarkerShape=Sphere  MarkerSize=10  GraphicVisPropType=SimpleVisualProperties  GraphicDiffuseColor=[1.0 0.6 0.2]  GraphicSpecularColor=[0.5 0.5 0.5 1.0]  GraphicAmbientColor=[0.15 0.15 0.15 1.0]  GraphicEmissiveColor=[0.0 0.0 0.0 1.0]  GraphicShininess=75  GraphicOpacity=1.0
  Conn2 : PMIOPort  Side=Left
  Conn3 : PMIOPort  Port=2  Side=Right
  connections:
  Rigid Transform3/LConn1 -- link4/RConn1 -- Conn2/RConn1
  Rigid Transform3/RConn1 -- Conn3/RConn1

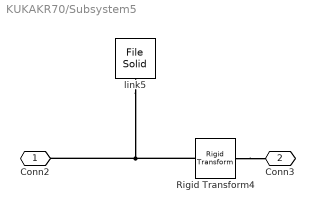
== system KUKAKR70/Subsystem5 ==
  Rigid Transform4 : sm_lib/Frames and Transforms/Rigid Transform  TranslationMethod=Cartesian  TranslationStandardOffset=0  TranslationLengthUnit=mm  TranslationStandardAxis=+Z  TranslationCartesianOffset=[0 -156.55 0]  TranslationROffset=0  TranslationROffsetUnits=m  TranslationZOffset=0  TranslationZOffsetUnits=m  TranslationThetaOffset=0  TranslationThetaOffsetUnits=deg  RotationMethod=RotationSequence  RotationAngleUnits=deg  RotationStandardAxis=+Z  RotationAngle=0.0  RotationArbitraryAxis=[0 0 1]  FollAlignAxisA=+X  BaseAlignAxisA=+Y  FollAlignAxisB=+Y  BaseAlignAxisB=+Z  RotationSequenceAxes=FollowerAxes  RotationSequence=XYZ  RotationSequenceAngles=[90 0 0]  RotationSequenceAnglesUnits=deg  RotationMatrix=[1 0 0; 0 1 0; 0 0 1]  Quaternion=[1 0 0 0]
  link5 : sm_lib/Body Elements/File Solid  ExtGeomFileName=C:\Users\revdu\OneDrive\Belgeler\GitHub\KukaKR70KinematicDynamicAnalysis\ComputedTorqueControl\stl\link5.stl  UnitType=Custom  ExtGeomFileUnits=mm  StepReaderType=HEX  ExportConvexHullGeometry=off  InertiaType=Custom  Mass=15.838  MassUnits=kg  CenterOfMass=[-0.08 -34.81 55.37]  CenterOfMassUnits=mm  MomentsOfInertia=[0.170 0.109 0.119]  MomentsOfInertiaUnits=kg*m^2  ProductsOfInertia=[0 0 -0.019]  ProductsOfInertiaUnits=kg*m^2  BasedOnType=DensityFromFile  Density=1000  DensityUnits=kg/m^3  DoExposeReferenceFrame=on  SerializedFrames=<Frames/>  GraphicType=FromGeometry  MarkerShape=Sphere  MarkerSize=10  GraphicVisPropType=SimpleVisualProperties  GraphicDiffuseColor=[0.4 0.4 0.4]  GraphicSpecularColor=[0.5 0.5 0.5 1.0]  GraphicAmbientColor=[0.15 0.15 0.15 1.0]  GraphicEmissiveColor=[0.0 0.0 0.0 1.0]  GraphicShininess=75  GraphicOpacity=1.0
  Conn2 : PMIOPort  Side=Left
  Conn3 : PMIOPort  Port=2  Side=Right
  connections:
  Rigid Transform4/LConn1 -- Conn2/RConn1 -- link5/RConn1
  Rigid Transform4/RConn1 -- Conn3/RConn1

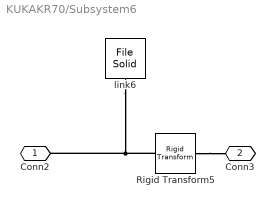
== system KUKAKR70/Subsystem6 ==
  Rigid Transform5 : sm_lib/Frames and Transforms/Rigid Transform  TranslationMethod=Cartesian  TranslationStandardOffset=0  TranslationLengthUnit=mm  TranslationStandardAxis=+Z  TranslationCartesianOffset=[0 0 30]  TranslationROffset=0  TranslationROffsetUnits=m  TranslationZOffset=0  TranslationZOffsetUnits=m  TranslationThetaOffset=0  TranslationThetaOffsetUnits=deg  RotationMethod=RotationSequence  RotationAngleUnits=deg  RotationStandardAxis=+Z  RotationAngle=0.0  RotationArbitraryAxis=[0 0 1]  FollAlignAxisA=+X  BaseAlignAxisA=+Y  FollAlignAxisB=+Y  BaseAlignAxisB=+Z  RotationSequenceAxes=FollowerAxes  RotationSequence=XYZ  RotationSequenceAngles=[0 0 0]  RotationSequenceAnglesUnits=deg  RotationMatrix=[1 0 0; 0 1 0; 0 0 1]  Quaternion=[1 0 0 0]
  link6 : sm_lib/Body Elements/File Solid  ExtGeomFileName=C:\Users\revdu\OneDrive\Belgeler\GitHub\KukaKR70KinematicDynamicAnalysis\ComputedTorqueControl\stl\link6.stl  UnitType=Custom  ExtGeomFileUnits=mm  StepReaderType=HEX  ExportConvexHullGeometry=off  InertiaType=Custom  Mass=1.111  MassUnits=kg  CenterOfMass=[-0.04 0 11.43]  CenterOfMassUnits=mm  MomentsOfInertia=[0.001 0.001 0.002]  MomentsOfInertiaUnits=kg*m^2  ProductsOfInertia=[0 0 0]  ProductsOfInertiaUnits=kg*m^2  BasedOnType=DensityFromFile  Density=1000  DensityUnits=kg/m^3  DoExposeReferenceFrame=on  SerializedFrames=<Frames/>  GraphicType=FromGeometry  MarkerShape=Sphere  MarkerSize=10  GraphicVisPropType=SimpleVisualProperties  GraphicDiffuseColor=[1.0 0.6 0.0]  GraphicSpecularColor=[0.5 0.5 0.5 1.0]  GraphicAmbientColor=[0.15 0.15 0.15 1.0]  GraphicEmissiveColor=[0.0 0.0 0.0 1.0]  GraphicShininess=75  GraphicOpacity=1.0
  Conn2 : PMIOPort  Side=Left
  Conn3 : PMIOPort  Port=2  Side=Right
  connections:
  Rigid Transform5/RConn1 -- Conn3/RConn1
  Rigid Transform5/LConn1 -- Conn2/RConn1 -- link6/RConn1

== matlab function KUKAKR70/MATLAB Function ==
  data: u input; y output
function y = fcn(u)

y = [u];
